simulink library "DblSlaveLib"  (R2020b)
settings: Solver=VariableStepAuto  StartTime=0.0  StopTime=10.0  RelTol=1e-3
libraries: simulink x7, InterpolationLib x4, $bdroot x3, Ramp_Library_R2017b x1
Description:
  | VLS Standard Library
  | Version: 1.0.0
settings Model: Creator=mchawa  LastModifiedBy=ahashem
settings DataIOCC: ReturnWorkspaceOutputs=off
settings DebuggingCC: ArithmeticOperatorsInVariantConditions=warning
settings SFSimCC: SimUseLocalCustomCode=off  CustomCodeUndefinedFunction=UseInterfaceOnly
settings RTWCC: RTWUseLocalCustomCode=off

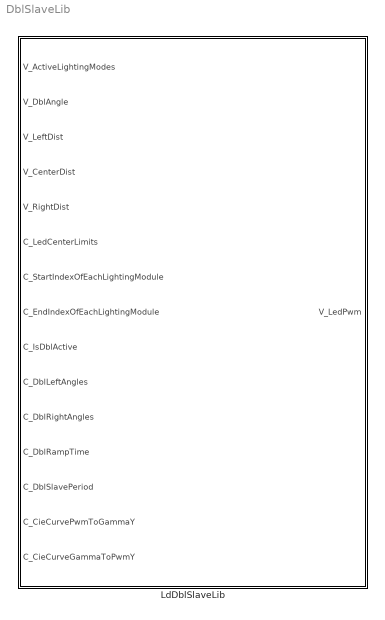
== system DblSlaveLib ==
  LdDblSlaveLib : Subsystem

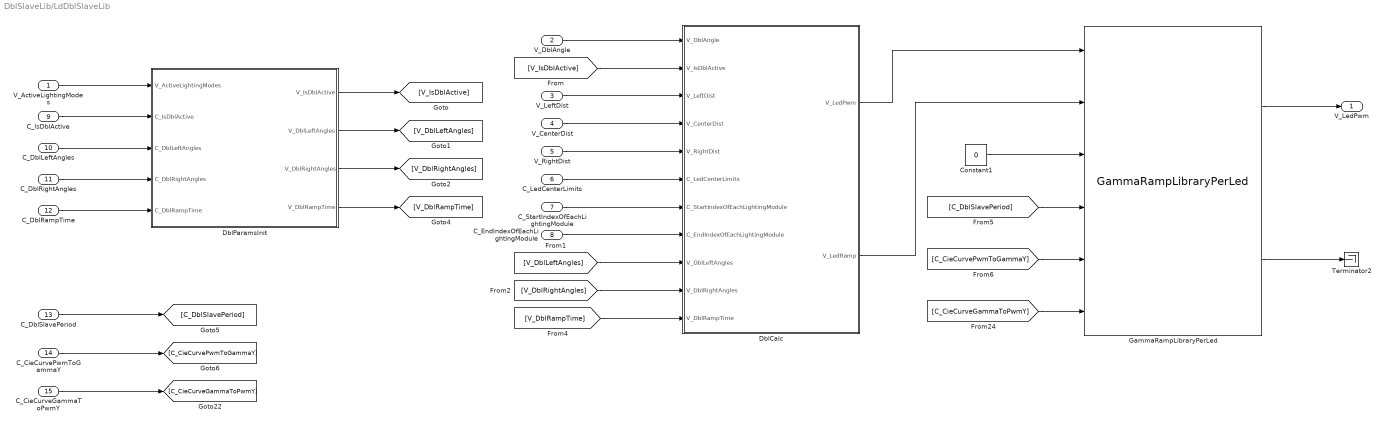
== system DblSlaveLib/LdDblSlaveLib ==
  V_ActiveLightingModes : Inport
  V_DblAngle : Inport  Port=2
  V_LeftDist : Inport  Port=3
  V_CenterDist : Inport  Port=4
  V_RightDist : Inport  Port=5
  C_LedCenterLimits : Inport  Port=6
  C_StartIndexOfEachLightingModule : Inport  Port=7
  C_EndIndexOfEachLightingModule : Inport  Port=8
  C_IsDblActive : Inport  Port=9
  C_DblLeftAngles : Inport  Port=10
  C_DblRightAngles : Inport  Port=11
  C_DblRampTime : Inport  Port=12
  C_DblSlavePeriod : Inport  Port=13
  C_CieCurvePwmToGammaY : Inport  Port=14
  C_CieCurveGammaToPwmY : Inport  Port=15
  Constant1 : Constant  Value=0  OutDataTypeStr=uint8
  DblCalc : Subsystem  TreatAsAtomicUnit=on
  DblParamsInit : Subsystem  TreatAsAtomicUnit=on
  GammaRampLibraryPerLed : Ramp_Library_R2017b/GammaRampLibraryPerLed  Description=|  SystemSampleTime=-1  VariantActivationTime=update diagram  Latency=0  AutoFrameSizeCalculation=off
      | This library performs ramp function taking CIE curves which are evenly distributed.
      | It performs the ramp linearly on the Gamma Curve.
  Terminator2 : Terminator
  V_LedPwm : Outport  VectorParamsAs1DForOutWhenUnconnected=off
  wires:
  C_EndIndexOfEachLightingModule/1 -> DblCalc/8(C_EndIndexOfEachLightingModule)
  DblParamsInit/1(V_IsDblActive) -> [V_IsDblActive]
  DblParamsInit/2(V_DblLeftAngles) -> [V_DblLeftAngles]
  [V_DblLeftAngles] -> DblCalc/9(V_DblLeftAngles)
  [V_DblRightAngles] -> DblCalc/10(V_DblRightAngles)
  C_LedCenterLimits/1 -> DblCalc/6(C_LedCenterLimits)
  DblParamsInit/3(V_DblRightAngles) -> [V_DblRightAngles]
  V_DblAngle/1 -> DblCalc/1(V_DblAngle)
  [V_IsDblActive] -> DblCalc/2(V_IsDblActive)
  C_StartIndexOfEachLightingModule/1 -> DblCalc/7(C_StartIndexOfEachLightingModule)
  GammaRampLibraryPerLed/1 -> V_LedPwm/1
  V_ActiveLightingModes/1 -> DblParamsInit/1(V_ActiveLightingModes)
  V_LeftDist/1 -> DblCalc/3(V_LeftDist)
  V_RightDist/1 -> DblCalc/5(V_RightDist)
  C_IsDblActive/1 -> DblParamsInit/2(C_IsDblActive)
  C_DblRampTime/1 -> DblParamsInit/5(C_DblRampTime)
  DblParamsInit/4(V_DblRampTime) -> [V_DblRampTime]
  C_DblLeftAngles/1 -> DblParamsInit/3(C_DblLeftAngles)
  V_CenterDist/1 -> DblCalc/4(V_CenterDist)
  C_DblRightAngles/1 -> DblParamsInit/4(C_DblRightAngles)
  DblCalc/1(V_LedPwm) -> GammaRampLibraryPerLed/1
  Constant1/1 -> GammaRampLibraryPerLed/3
  GammaRampLibraryPerLed/2 -> Terminator2/1
  C_CieCurveGammaToPwmY/1 -> [C_CieCurveGammaToPwmY]
  C_CieCurvePwmToGammaY/1 -> [C_CieCurvePwmToGammaY]
  C_DblSlavePeriod/1 -> [C_DblSlavePeriod]
  [C_CieCurveGammaToPwmY] -> GammaRampLibraryPerLed/6
  [C_CieCurvePwmToGammaY] -> GammaRampLibraryPerLed/5
  [C_DblSlavePeriod] -> GammaRampLibraryPerLed/4
  [V_DblRampTime] -> DblCalc/11(V_DblRampTime)
  DblCalc/2(V_LedRamp) -> GammaRampLibraryPerLed/2

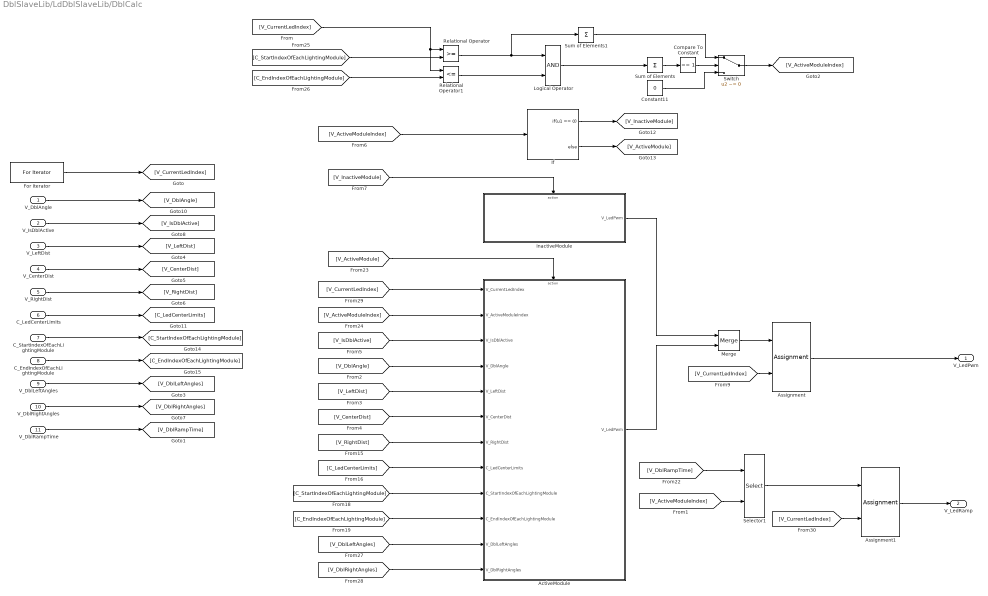
== system DblSlaveLib/LdDblSlaveLib/DblCalc ==
  V_DblAngle : Inport
  V_IsDblActive : Inport  Port=2
  V_LeftDist : Inport  Port=3
  V_CenterDist : Inport  Port=4
  V_RightDist : Inport  Port=5
  C_LedCenterLimits : Inport  Port=6
  C_StartIndexOfEachLightingModule : Inport  Port=7
  C_EndIndexOfEachLightingModule : Inport  Port=8
  V_DblLeftAngles : Inport  Port=9
  V_DblRightAngles : Inport  Port=10
  V_DblRampTime : Inport  Port=11
  ActiveModule : Subsystem  TreatAsAtomicUnit=on
  Assignment : Assignment  IndexMode=Zero-based  OutputInitialize=Specify size for each dimension in table  DiagnosticForDimensions=Error  IndexOptions=Index vector (port)  Indices=1  OutputSizes=C_NumOfLightingLeds
  Assignment1 : Assignment  IndexMode=Zero-based  OutputInitialize=Specify size for each dimension in table  DiagnosticForDimensions=Error  IndexOptions=Index vector (port)  Indices=1  OutputSizes=C_NumOfLightingLeds
  Compare To Constant : simulink/Logic and Bit Operations/Compare To Constant  relop===  const=1  OutDataTypeStr=boolean
  Constant11 : Constant  Value=0  OutDataTypeStr=Inherit: Inherit via back propagation
  For Iterator : ForIterator  IterationLimit=C_NumOfLightingLeds  IndexMode=Zero-based
  If : If  IfExpression=u1 == 0
  InactiveModule : Subsystem  TreatAsAtomicUnit=on
  Logical Operator : Logic  AllPortsSameDT=off  OutDataTypeStr=boolean
  Merge : Merge
  Relational Operator : RelationalOperator  OutDataTypeStr=boolean  RndMeth=Simplest
  Relational Operator1 : RelationalOperator  Operator=<=  OutDataTypeStr=boolean  RndMeth=Simplest
  Selector1 : Selector  IndexOptions=Index vector (port)  Indices=[1 3]  OutputSizes=1
  Sum of Elements : Sum  Inputs=+
  Sum of Elements1 : Sum  Inputs=+
  Switch : Switch  Criteria=u2 ~= 0
  V_LedPwm : Outport  VectorParamsAs1DForOutWhenUnconnected=off
  V_LedRamp : Outport  Port=2  VectorParamsAs1DForOutWhenUnconnected=off
  wires:
  For Iterator/1 -> [V_CurrentLedIndex]
  [V_CurrentLedIndex] -> Relational Operator/1, Relational Operator1/1
  V_LeftDist/1 -> [V_LeftDist]
  V_CenterDist/1 -> [V_CenterDist]
  V_RightDist/1 -> [V_RightDist]
  V_DblAngle/1 -> [V_DblAngle]
  Assignment/1 -> V_LedPwm/1
  [V_CurrentLedIndex] -> Assignment/2
  Relational Operator/1 -> Sum of Elements1/1, Logical Operator/1
  Logical Operator/1 -> Sum of Elements/1
  Relational Operator1/1 -> Logical Operator/2
  Sum of Elements/1 -> Compare To Constant/1
  Switch/1 -> [V_ActiveModuleIndex]
  Constant11/1 -> Switch/3
  Sum of Elements1/1 -> Switch/1
  Compare To Constant/1 -> Switch/2
  C_LedCenterLimits/1 -> [C_LedCenterLimits]
  [V_ActiveModuleIndex] -> If/1
  If/1 -> [V_InactiveModule]
  If/2 -> [V_ActiveModule]
  [V_InactiveModule] -> InactiveModule/Action
  [V_ActiveModule] -> ActiveModule/Action
  [V_ActiveModuleIndex] -> ActiveModule/2(V_ActiveModuleIndex)
  C_StartIndexOfEachLightingModule/1 -> [C_StartIndexOfEachLightingModule]
  C_EndIndexOfEachLightingModule/1 -> [C_EndIndexOfEachLightingModule]
  [C_StartIndexOfEachLightingModule] -> Relational Operator/2
  [C_EndIndexOfEachLightingModule] -> Relational Operator1/2
  ActiveModule/1(V_LedPwm) -> Merge/2
  InactiveModule/1(V_LedPwm) -> Merge/1
  Merge/1 -> Assignment/1
  V_DblLeftAngles/1 -> [V_DblLeftAngles]
  V_DblRightAngles/1 -> [V_DblRightAngles]
  [V_DblAngle] -> ActiveModule/4(V_DblAngle)
  [V_LeftDist] -> ActiveModule/5(V_LeftDist)
  [V_CenterDist] -> ActiveModule/6(V_CenterDist)
  [V_RightDist] -> ActiveModule/7(V_RightDist)
  [C_LedCenterLimits] -> ActiveModule/8(C_LedCenterLimits)
  [C_StartIndexOfEachLightingModule] -> ActiveModule/9(C_StartIndexOfEachLightingModule)
  [C_EndIndexOfEachLightingModule] -> ActiveModule/10(C_EndIndexOfEachLightingModule)
  [V_DblLeftAngles] -> ActiveModule/11(V_DblLeftAngles)
  [V_DblRightAngles] -> ActiveModule/12(V_DblRightAngles)
  [V_CurrentLedIndex] -> ActiveModule/1(V_CurrentLedIndex)
  V_IsDblActive/1 -> [V_IsDblActive]
  [V_IsDblActive] -> ActiveModule/3(V_IsDblActive)
  V_DblRampTime/1 -> [V_DblRampTime]
  Selector1/1 -> Assignment1/1
  [V_CurrentLedIndex] -> Assignment1/2
  Assignment1/1 -> V_LedRamp/1
  [V_DblRampTime] -> Selector1/1
  [V_ActiveModuleIndex] -> Selector1/2

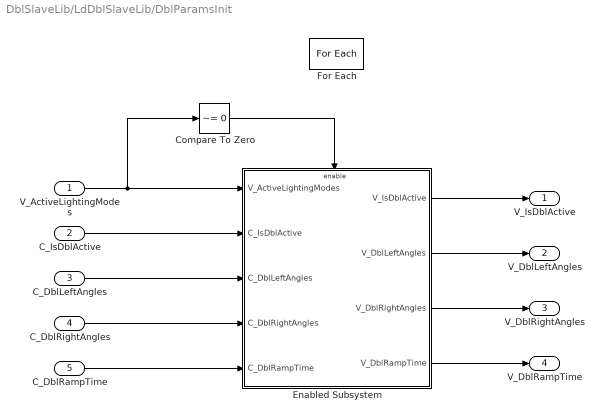
== system DblSlaveLib/LdDblSlaveLib/DblParamsInit ==
  V_ActiveLightingModes : Inport  Partition=on  PartitionDimension=1  PartitionWidth=1  PartitionOffset=0
  C_IsDblActive : Inport  Port=2  Partition=on  PartitionDimension=1  PartitionWidth=1  PartitionOffset=0
  C_DblLeftAngles : Inport  Port=3  Partition=on  PartitionDimension=1  PartitionWidth=1  PartitionOffset=0
  C_DblRightAngles : Inport  Port=4  Partition=on  PartitionDimension=1  PartitionWidth=1  PartitionOffset=0
  C_DblRampTime : Inport  Port=5  Partition=on  PartitionDimension=1  PartitionWidth=1  PartitionOffset=0
  Compare To Zero : simulink/Logic and Bit Operations/Compare To Zero  relop=~=  OutDataTypeStr=boolean
  Enabled Subsystem : Subsystem  TreatAsAtomicUnit=on
  For Each : ForEach  DisableCoverage=on
  V_IsDblActive : Outport  ConcatenationDimension=1  VectorParamsAs1DForOutWhenUnconnected=off
  V_DblLeftAngles : Outport  Port=2  ConcatenationDimension=1  VectorParamsAs1DForOutWhenUnconnected=off
  V_DblRightAngles : Outport  Port=3  ConcatenationDimension=1  VectorParamsAs1DForOutWhenUnconnected=off
  V_DblRampTime : Outport  Port=4  ConcatenationDimension=1  VectorParamsAs1DForOutWhenUnconnected=off
  wires:
  Compare To Zero/1 -> Enabled Subsystem/Enable
  V_ActiveLightingModes/1 -> Compare To Zero/1, Enabled Subsystem/1(V_ActiveLightingModes)
  C_IsDblActive/1 -> Enabled Subsystem/2(C_IsDblActive)
  Enabled Subsystem/1(V_IsDblActive) -> V_IsDblActive/1
  C_DblLeftAngles/1 -> Enabled Subsystem/3(C_DblLeftAngles)
  C_DblRightAngles/1 -> Enabled Subsystem/4(C_DblRightAngles)
  Enabled Subsystem/3(V_DblRightAngles) -> V_DblRightAngles/1
  Enabled Subsystem/2(V_DblLeftAngles) -> V_DblLeftAngles/1
  C_DblRampTime/1 -> Enabled Subsystem/5(C_DblRampTime)
  Enabled Subsystem/4(V_DblRampTime) -> V_DblRampTime/1

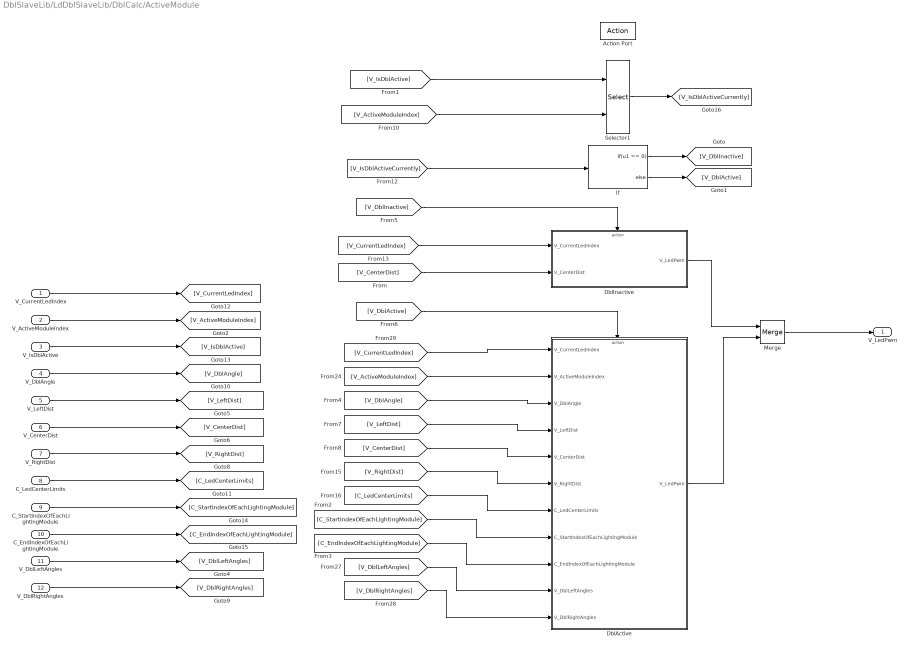
== system DblSlaveLib/LdDblSlaveLib/DblCalc/ActiveModule ==
  V_CurrentLedIndex : Inport
  V_ActiveModuleIndex : Inport  Port=2
  V_IsDblActive : Inport  Port=3
  V_DblAngle : Inport  Port=4
  V_LeftDist : Inport  Port=5
  V_CenterDist : Inport  Port=6
  V_RightDist : Inport  Port=7
  C_LedCenterLimits : Inport  Port=8
  C_StartIndexOfEachLightingModule : Inport  Port=9
  C_EndIndexOfEachLightingModule : Inport  Port=10
  V_DblLeftAngles : Inport  Port=11
  V_DblRightAngles : Inport  Port=12
  Action Port : ActionPort
  DblActive : Subsystem  TreatAsAtomicUnit=on
  DblInactive : Subsystem  TreatAsAtomicUnit=on
  If : If  IfExpression=u1 == 0
  Merge : Merge
  Selector1 : Selector  IndexOptions=Index vector (port)  Indices=[1 3]  OutputSizes=1
  V_LedPwm : Outport  VectorParamsAs1DForOutWhenUnconnected=off
  wires:
  [V_IsDblActiveCurrently] -> If/1
  If/1 -> [V_DblInactive]
  If/2 -> [V_DblActive]
  [V_DblInactive] -> DblInactive/Action
  [V_DblActive] -> DblActive/Action
  DblActive/1(V_LedPwm) -> Merge/2
  DblInactive/1(V_LedPwm) -> Merge/1
  Merge/1 -> V_LedPwm/1
  V_ActiveModuleIndex/1 -> [V_ActiveModuleIndex]
  V_DblAngle/1 -> [V_DblAngle]
  V_LeftDist/1 -> [V_LeftDist]
  V_CenterDist/1 -> [V_CenterDist]
  V_RightDist/1 -> [V_RightDist]
  C_LedCenterLimits/1 -> [C_LedCenterLimits]
  C_StartIndexOfEachLightingModule/1 -> [C_StartIndexOfEachLightingModule]
  C_EndIndexOfEachLightingModule/1 -> [C_EndIndexOfEachLightingModule]
  V_DblLeftAngles/1 -> [V_DblLeftAngles]
  V_DblRightAngles/1 -> [V_DblRightAngles]
  V_CurrentLedIndex/1 -> [V_CurrentLedIndex]
  [V_CurrentLedIndex] -> DblActive/1(V_CurrentLedIndex)
  [V_ActiveModuleIndex] -> DblActive/2(V_ActiveModuleIndex)
  [V_DblAngle] -> DblActive/3(V_DblAngle)
  [V_LeftDist] -> DblActive/4(V_LeftDist)
  [V_CenterDist] -> DblActive/5(V_CenterDist)
  [V_RightDist] -> DblActive/6(V_RightDist)
  [C_LedCenterLimits] -> DblActive/7(C_LedCenterLimits)
  [C_StartIndexOfEachLightingModule] -> DblActive/8(C_StartIndexOfEachLightingModule)
  [C_EndIndexOfEachLightingModule] -> DblActive/9(C_EndIndexOfEachLightingModule)
  [V_DblLeftAngles] -> DblActive/10(V_DblLeftAngles)
  [V_DblRightAngles] -> DblActive/11(V_DblRightAngles)
  V_IsDblActive/1 -> [V_IsDblActive]
  [V_IsDblActive] -> Selector1/1
  [V_ActiveModuleIndex] -> Selector1/2
  Selector1/1 -> [V_IsDblActiveCurrently]
  [V_CenterDist] -> DblInactive/2(V_CenterDist)
  [V_CurrentLedIndex] -> DblInactive/1(V_CurrentLedIndex)

== system DblSlaveLib/LdDblSlaveLib/DblCalc/InactiveModule ==
  Action Port : ActionPort
  Constant : Constant  Value=0  OutDataTypeStr=Inherit: Inherit via back propagation
  V_LedPwm : Outport  VectorParamsAs1DForOutWhenUnconnected=off
  wires:
  Constant/1 -> V_LedPwm/1

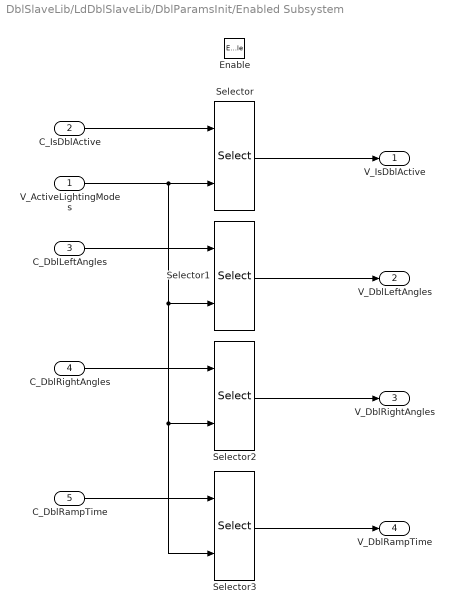
== system DblSlaveLib/LdDblSlaveLib/DblParamsInit/Enabled Subsystem ==
  V_ActiveLightingModes : Inport
  C_IsDblActive : Inport  Port=2
  C_DblLeftAngles : Inport  Port=3
  C_DblRightAngles : Inport  Port=4
  C_DblRampTime : Inport  Port=5
  Enable : EnablePort
  Selector{,1..3} (4 alike) : Selector  IndexOptions=Index vector (port)  Indices=[1 3]  OutputSizes=1
  V_IsDblActive : Outport  VectorParamsAs1DForOutWhenUnconnected=off
  V_DblLeftAngles : Outport  Port=2  VectorParamsAs1DForOutWhenUnconnected=off
  V_DblRightAngles : Outport  Port=3  VectorParamsAs1DForOutWhenUnconnected=off
  V_DblRampTime : Outport  Port=4  VectorParamsAs1DForOutWhenUnconnected=off
  wires:
  Selector/1 -> V_IsDblActive/1
  C_IsDblActive/1 -> Selector/1
  V_ActiveLightingModes/1 -> Selector3/2, Selector2/2, Selector1/2, Selector/2
  C_DblLeftAngles/1 -> Selector1/1
  C_DblRightAngles/1 -> Selector2/1
  Selector1/1 -> V_DblLeftAngles/1
  Selector2/1 -> V_DblRightAngles/1
  C_DblRampTime/1 -> Selector3/1
  Selector3/1 -> V_DblRampTime/1

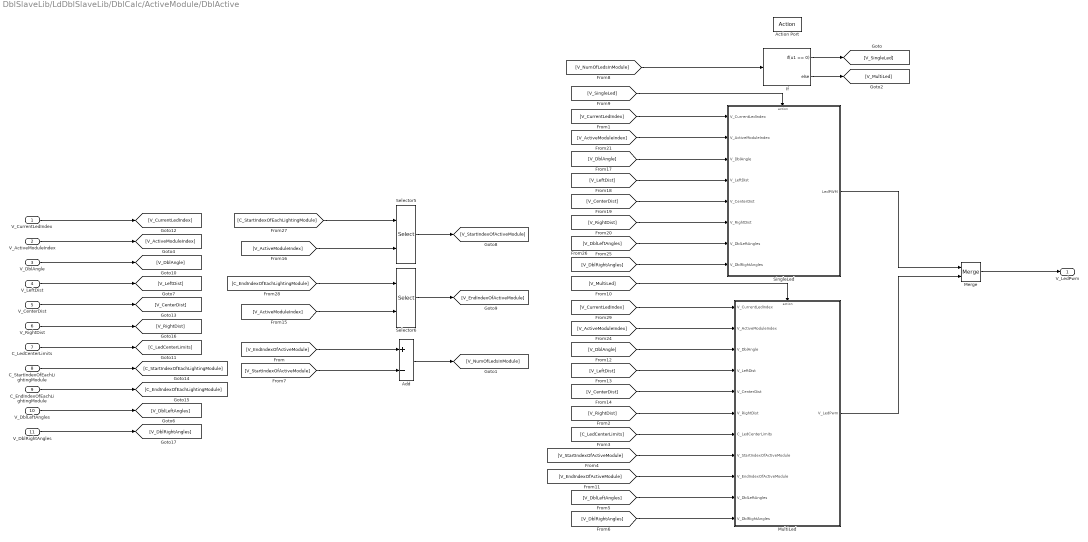
== system DblSlaveLib/LdDblSlaveLib/DblCalc/ActiveModule/DblActive ==
  V_CurrentLedIndex : Inport
  V_ActiveModuleIndex : Inport  Port=2
  V_DblAngle : Inport  Port=3
  V_LeftDist : Inport  Port=4
  V_CenterDist : Inport  Port=5
  V_RightDist : Inport  Port=6
  C_LedCenterLimits : Inport  Port=7
  C_StartIndexOfEachLightingModule : Inport  Port=8
  C_EndIndexOfEachLightingModule : Inport  Port=9
  V_DblLeftAngles : Inport  Port=10
  V_DblRightAngles : Inport  Port=11
  Action Port : ActionPort
  Add : Sum  Inputs=+-
  If : If  IfExpression=u1 == 0
  Merge : Merge
  MultiLed : Subsystem  TreatAsAtomicUnit=on
  Selector5 : Selector  IndexOptions=Index vector (port)  Indices=[1 3]  OutputSizes=1
  Selector6 : Selector  IndexOptions=Index vector (port)  Indices=[1 3]  OutputSizes=1
  SingleLed : Subsystem  TreatAsAtomicUnit=on
  V_LedPwm : Outport  VectorParamsAs1DForOutWhenUnconnected=off
  wires:
  [V_ActiveModuleIndex] -> Selector5/2
  [C_EndIndexOfEachLightingModule] -> Selector6/1
  [V_ActiveModuleIndex] -> Selector6/2
  Selector6/1 -> [V_EndIndexOfActiveModule]
  [C_StartIndexOfEachLightingModule] -> Selector5/1
  Selector5/1 -> [V_StartIndexOfActiveModule]
  [V_EndIndexOfActiveModule] -> Add/1
  [V_StartIndexOfActiveModule] -> Add/2
  Add/1 -> [V_NumOfLedsInModule]
  [V_NumOfLedsInModule] -> If/1
  If/1 -> [V_SingleLed]
  If/2 -> [V_MultiLed]
  [V_SingleLed] -> SingleLed/Action
  [V_MultiLed] -> MultiLed/Action
  MultiLed/1(V_LedPwm) -> Merge/2
  Merge/1 -> V_LedPwm/1
  V_CurrentLedIndex/1 -> [V_CurrentLedIndex]
  V_ActiveModuleIndex/1 -> [V_ActiveModuleIndex]
  V_DblAngle/1 -> [V_DblAngle]
  V_LeftDist/1 -> [V_LeftDist]
  V_CenterDist/1 -> [V_CenterDist]
  V_RightDist/1 -> [V_RightDist]
  C_LedCenterLimits/1 -> [C_LedCenterLimits]
  C_StartIndexOfEachLightingModule/1 -> [C_StartIndexOfEachLightingModule]
  C_EndIndexOfEachLightingModule/1 -> [C_EndIndexOfEachLightingModule]
  V_DblLeftAngles/1 -> [V_DblLeftAngles]
  V_DblRightAngles/1 -> [V_DblRightAngles]
  [V_CurrentLedIndex] -> MultiLed/1(V_CurrentLedIndex)
  [V_ActiveModuleIndex] -> MultiLed/2(V_ActiveModuleIndex)
  [V_LeftDist] -> MultiLed/4(V_LeftDist)
  [V_CenterDist] -> MultiLed/5(V_CenterDist)
  [V_RightDist] -> MultiLed/6(V_RightDist)
  [C_LedCenterLimits] -> MultiLed/7(C_LedCenterLimits)
  [V_StartIndexOfActiveModule] -> MultiLed/8(V_StartIndexOfActiveModule)
  [V_EndIndexOfActiveModule] -> MultiLed/9(V_EndIndexOfActiveModule)
  [V_DblLeftAngles] -> MultiLed/10(V_DblLeftAngles)
  [V_DblRightAngles] -> MultiLed/11(V_DblRightAngles)
  [V_DblAngle] -> MultiLed/3(V_DblAngle)
  [V_DblRightAngles] -> SingleLed/8(V_DblRightAngles)
  [V_LeftDist] -> SingleLed/4(V_LeftDist)
  [V_DblAngle] -> SingleLed/3(V_DblAngle)
  [V_DblLeftAngles] -> SingleLed/7(V_DblLeftAngles)
  [V_ActiveModuleIndex] -> SingleLed/2(V_ActiveModuleIndex)
  [V_RightDist] -> SingleLed/6(V_RightDist)
  [V_CenterDist] -> SingleLed/5(V_CenterDist)
  SingleLed/1(LedPWM) -> Merge/1
  [V_CurrentLedIndex] -> SingleLed/1(V_CurrentLedIndex)

== system DblSlaveLib/LdDblSlaveLib/DblCalc/ActiveModule/DblInactive ==
  V_CurrentLedIndex : Inport
  V_CenterDist : Inport  Port=2
  Action Port : ActionPort
  Selector : Selector  IndexMode=Zero-based  IndexOptions=Index vector (port)  Indices=[1 3]  OutputSizes=1
  V_LedPwm : Outport  VectorParamsAs1DForOutWhenUnconnected=off
  wires:
  V_CenterDist/1 -> Selector/1
  V_CurrentLedIndex/1 -> Selector/2
  Selector/1 -> V_LedPwm/1

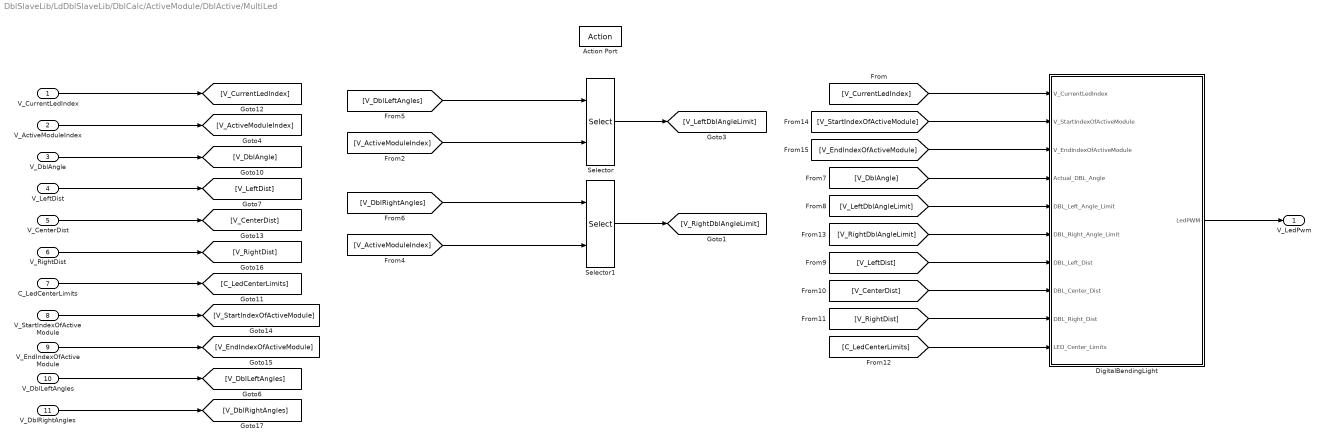
== system DblSlaveLib/LdDblSlaveLib/DblCalc/ActiveModule/DblActive/MultiLed ==
  V_CurrentLedIndex : Inport
  V_ActiveModuleIndex : Inport  Port=2
  V_DblAngle : Inport  Port=3
  V_LeftDist : Inport  Port=4
  V_CenterDist : Inport  Port=5
  V_RightDist : Inport  Port=6
  C_LedCenterLimits : Inport  Port=7
  V_StartIndexOfActiveModule : Inport  Port=8
  V_EndIndexOfActiveModule : Inport  Port=9
  V_DblLeftAngles : Inport  Port=10
  V_DblRightAngles : Inport  Port=11
  Action Port : ActionPort
  DigitalBendingLight : Subsystem  Description=|  TreatAsAtomicUnit=on
      | This block performs DBL function assuming that the DBL Left/Center/Right Distribution are of the same size as LED_Center_Limits.
      | Left DBL_Angles must be always less than Right DBL_Angles.
  Selector : Selector  IndexOptions=Index vector (port)  Indices=[1 3]  OutputSizes=1
  Selector1 : Selector  IndexOptions=Index vector (port)  Indices=[1 3]  OutputSizes=1
  V_LedPwm : Outport  VectorParamsAs1DForOutWhenUnconnected=off
  wires:
  [V_ActiveModuleIndex] -> Selector1/2
  [V_DblRightAngles] -> Selector1/1
  [V_DblLeftAngles] -> Selector/1
  [V_ActiveModuleIndex] -> Selector/2
  DigitalBendingLight/1(LedPWM) -> V_LedPwm/1
  V_ActiveModuleIndex/1 -> [V_ActiveModuleIndex]
  V_DblAngle/1 -> [V_DblAngle]
  V_DblLeftAngles/1 -> [V_DblLeftAngles]
  V_RightDist/1 -> [V_RightDist]
  V_DblRightAngles/1 -> [V_DblRightAngles]
  V_EndIndexOfActiveModule/1 -> [V_EndIndexOfActiveModule]
  V_LeftDist/1 -> [V_LeftDist]
  V_StartIndexOfActiveModule/1 -> [V_StartIndexOfActiveModule]
  C_LedCenterLimits/1 -> [C_LedCenterLimits]
  V_CurrentLedIndex/1 -> [V_CurrentLedIndex]
  V_CenterDist/1 -> [V_CenterDist]
  [V_CurrentLedIndex] -> DigitalBendingLight/1(V_CurrentLedIndex)
  [V_DblAngle] -> DigitalBendingLight/4(Actual_DBL_Angle)
  [V_LeftDblAngleLimit] -> DigitalBendingLight/5(DBL_Left_Angle_Limit)
  [V_LeftDist] -> DigitalBendingLight/7(DBL_Left_Dist)
  [V_CenterDist] -> DigitalBendingLight/8(DBL_Center_Dist)
  [V_RightDist] -> DigitalBendingLight/9(DBL_Right_Dist)
  [C_LedCenterLimits] -> DigitalBendingLight/10(LED_Center_Limits)
  Selector/1 -> [V_LeftDblAngleLimit]
  Selector1/1 -> [V_RightDblAngleLimit]
  [V_RightDblAngleLimit] -> DigitalBendingLight/6(DBL_Right_Angle_Limit)
  [V_StartIndexOfActiveModule] -> DigitalBendingLight/2(V_StartIndexOfActiveModule)
  [V_EndIndexOfActiveModule] -> DigitalBendingLight/3(V_EndIndexOfActiveModule)

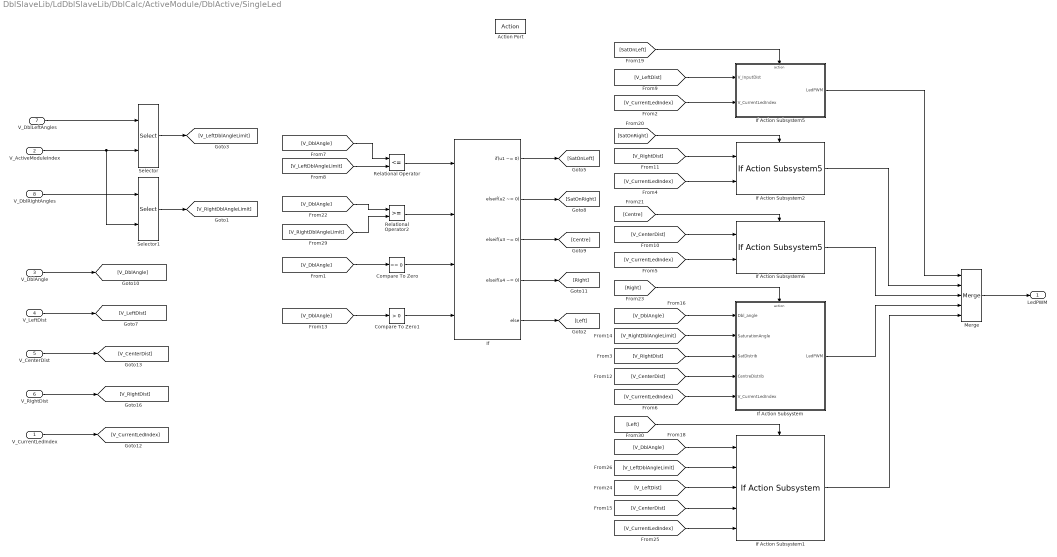
== system DblSlaveLib/LdDblSlaveLib/DblCalc/ActiveModule/DblActive/SingleLed ==
  V_CurrentLedIndex : Inport
  V_ActiveModuleIndex : Inport  Port=2
  V_DblAngle : Inport  Port=3
  V_LeftDist : Inport  Port=4
  V_CenterDist : Inport  Port=5
  V_RightDist : Inport  Port=6
  V_DblLeftAngles : Inport  Port=7
  V_DblRightAngles : Inport  Port=8
  Action Port : ActionPort
  Compare To Zero : simulink/Logic and Bit Operations/Compare To Zero  relop===  OutDataTypeStr=boolean
  Compare To Zero1 : simulink/Logic and Bit Operations/Compare To Zero  relop=>  OutDataTypeStr=boolean
  If : If  NumInputs=4  IfExpression=u1 ~= 0  ElseIfExpressions=u2 ~= 0, u3 ~= 0,u4 ~= 0
  If Action Subsystem : Subsystem  TreatAsAtomicUnit=on
  If Action Subsystem1 : $bdroot/LdDblSlaveLib/DblCalc/ActiveModule/DblActive/SingleLed/If Action Subsystem  SystemSampleTime=-1  VariantActivationTime=update diagram  Latency=0  AutoFrameSizeCalculation=off
  If Action Subsystem2 : $bdroot/LdDblSlaveLib/DblCalc/ActiveModule/DblActive/SingleLed/If Action Subsystem5  SystemSampleTime=-1  VariantActivationTime=update diagram  Latency=0  AutoFrameSizeCalculation=off
  If Action Subsystem5 : Subsystem  TreatAsAtomicUnit=on
  If Action Subsystem6 : $bdroot/LdDblSlaveLib/DblCalc/ActiveModule/DblActive/SingleLed/If Action Subsystem5  SystemSampleTime=-1  VariantActivationTime=update diagram  Latency=0  AutoFrameSizeCalculation=off
  Merge : Merge  Inputs=5  InitialOutput=0
  Relational Operator : RelationalOperator  Operator=<=  OutDataTypeStr=boolean  RndMeth=Simplest
  Relational Operator2 : RelationalOperator  OutDataTypeStr=boolean  RndMeth=Simplest
  Selector : Selector  IndexOptions=Index vector (port)  Indices=[1 3]  OutputSizes=1
  Selector1 : Selector  IndexOptions=Index vector (port)  Indices=[1 3]  OutputSizes=1
  LedPWM : Outport  VectorParamsAs1DForOutWhenUnconnected=off
  wires:
  V_DblRightAngles/1 -> Selector1/1
  V_DblLeftAngles/1 -> Selector/1
  Selector1/1 -> [V_RightDblAngleLimit]
  Selector/1 -> [V_LeftDblAngleLimit]
  V_ActiveModuleIndex/1 -> Selector/2, Selector1/2
  V_DblAngle/1 -> [V_DblAngle]
  V_LeftDist/1 -> [V_LeftDist]
  V_RightDist/1 -> [V_RightDist]
  V_CenterDist/1 -> [V_CenterDist]
  Relational Operator2/1 -> If/2
  Compare To Zero/1 -> If/3
  If/3 -> [Centre]
  [SatOnLeft] -> If Action Subsystem5/Action
  [V_CenterDist] -> If Action Subsystem6/1
  [Centre] -> If Action Subsystem6/Action
  Merge/1 -> LedPWM/1
  If/2 -> [SatOnRight]
  If/1 -> [SatOnLeft]
  Relational Operator/1 -> If/1
  [V_DblAngle] -> Compare To Zero/1
  [Right] -> If Action Subsystem/Action
  [V_DblAngle] -> Relational Operator2/1
  If/5 -> [Left]
  [V_RightDblAngleLimit] -> Relational Operator2/2
  [V_LeftDblAngleLimit] -> Relational Operator/2
  [V_DblAngle] -> Relational Operator/1
  Compare To Zero1/1 -> If/4
  [V_DblAngle] -> Compare To Zero1/1
  If/4 -> [Right]
  [Left] -> If Action Subsystem1/Action
  [V_RightDist] -> If Action Subsystem/3(SatDistrib)
  [V_CenterDist] -> If Action Subsystem/4(CentreDistrib)
  [V_RightDblAngleLimit] -> If Action Subsystem/2(SaturationAngle)
  [SatOnRight] -> If Action Subsystem2/Action
  [V_RightDist] -> If Action Subsystem2/1
  [V_DblAngle] -> If Action Subsystem/1(Dbl_angle)
  [V_DblAngle] -> If Action Subsystem1/1
  [V_LeftDblAngleLimit] -> If Action Subsystem1/2
  [V_CenterDist] -> If Action Subsystem1/4
  [V_LeftDist] -> If Action Subsystem1/3
  If Action Subsystem5/1(LedPWM) -> Merge/1
  If Action Subsystem2/1 -> Merge/2
  If Action Subsystem6/1 -> Merge/3
  If Action Subsystem/1(LedPWM) -> Merge/4
  If Action Subsystem1/1 -> Merge/5
  [V_LeftDist] -> If Action Subsystem5/1(V_InputDist)
  [V_CurrentLedIndex] -> If Action Subsystem5/2(V_CurrentLedIndex)
  V_CurrentLedIndex/1 -> [V_CurrentLedIndex]
  [V_CurrentLedIndex] -> If Action Subsystem2/2
  [V_CurrentLedIndex] -> If Action Subsystem6/2
  [V_CurrentLedIndex] -> If Action Subsystem/5(V_CurrentLedIndex)
  [V_CurrentLedIndex] -> If Action Subsystem1/5

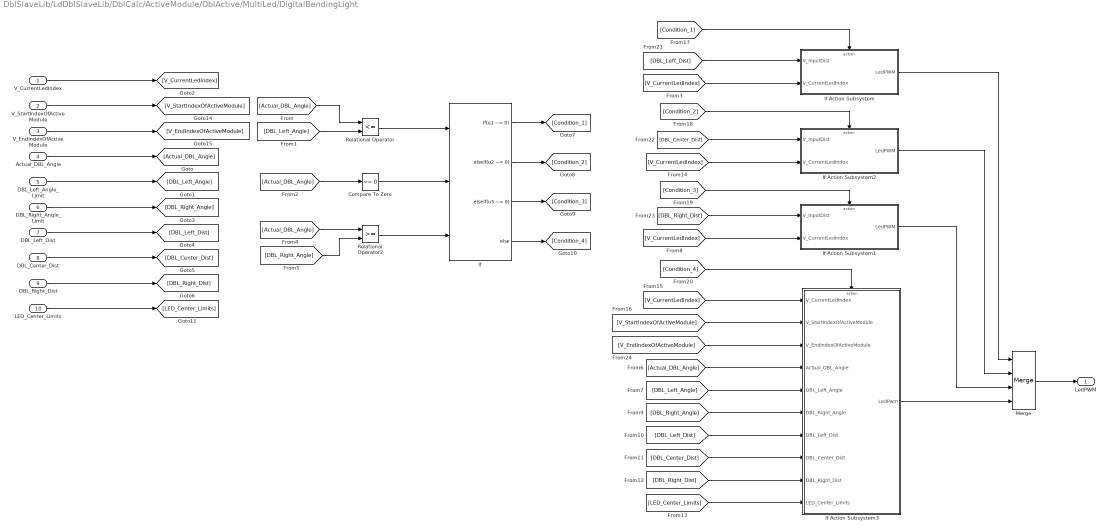
== system DblSlaveLib/LdDblSlaveLib/DblCalc/ActiveModule/DblActive/MultiLed/DigitalBendingLight ==
  V_CurrentLedIndex : Inport
  V_StartIndexOfActiveModule : Inport  Port=2
  V_EndIndexOfActiveModule : Inport  Port=3
  Actual_DBL_Angle : Inport  Port=4
  DBL_Left_Angle_Limit : Inport  Port=5
  DBL_Right_Angle_Limit : Inport  Port=6
  DBL_Left_Dist : Inport  Port=7
  DBL_Center_Dist : Inport  Port=8
  DBL_Right_Dist : Inport  Port=9
  LED_Center_Limits : Inport  Port=10
  Compare To Zero : simulink/Logic and Bit Operations/Compare To Zero  relop===  OutDataTypeStr=boolean
  If : If  NumInputs=3  IfExpression=u1 ~= 0  ElseIfExpressions=u2 ~= 0, u3 ~= 0
  If Action Subsystem : Subsystem  TreatAsAtomicUnit=on
  If Action Subsystem1 : Subsystem  TreatAsAtomicUnit=on
  If Action Subsystem2 : Subsystem  TreatAsAtomicUnit=on
  If Action Subsystem3 : Subsystem  TreatAsAtomicUnit=on
  Merge : Merge  Inputs=4  InitialOutput=0
  Relational Operator : RelationalOperator  Operator=<=  OutDataTypeStr=boolean  RndMeth=Simplest
  Relational Operator2 : RelationalOperator  OutDataTypeStr=boolean  RndMeth=Simplest
  LedPWM : Outport  VectorParamsAs1DForOutWhenUnconnected=off
  wires:
  Actual_DBL_Angle/1 -> [Actual_DBL_Angle]
  DBL_Left_Angle_Limit/1 -> [DBL_Left_Angle]
  DBL_Right_Angle_Limit/1 -> [DBL_Right_Angle]
  [Actual_DBL_Angle] -> Relational Operator/1
  [DBL_Left_Angle] -> Relational Operator/2
  [DBL_Right_Angle] -> Relational Operator2/2
  [Actual_DBL_Angle] -> Relational Operator2/1
  DBL_Left_Dist/1 -> [DBL_Left_Dist]
  DBL_Center_Dist/1 -> [DBL_Center_Dist]
  DBL_Right_Dist/1 -> [DBL_Right_Dist]
  Relational Operator/1 -> If/1
  [Actual_DBL_Angle] -> Compare To Zero/1
  Relational Operator2/1 -> If/3
  If/1 -> [Condition_1]
  If/2 -> [Condition_2]
  If/3 -> [Condition_3]
  [Condition_1] -> If Action Subsystem/Action
  [Condition_4] -> If Action Subsystem3/Action
  [DBL_Left_Dist] -> If Action Subsystem/1(V_InputDist)
  If/4 -> [Condition_4]
  [Actual_DBL_Angle] -> If Action Subsystem3/4(Actual_DBL_Angle)
  [DBL_Left_Angle] -> If Action Subsystem3/5(DBL_Left_Angle)
  [DBL_Right_Angle] -> If Action Subsystem3/6(DBL_Right_Angle)
  [DBL_Left_Dist] -> If Action Subsystem3/7(DBL_Left_Dist)
  [DBL_Center_Dist] -> If Action Subsystem3/8(DBL_Center_Dist)
  If Action Subsystem1/1(LedPWM) -> Merge/3
  If Action Subsystem2/1(LedPWM) -> Merge/2
  If Action Subsystem/1(LedPWM) -> Merge/1
  Merge/1 -> LedPWM/1
  [DBL_Right_Dist] -> If Action Subsystem3/9(DBL_Right_Dist)
  LED_Center_Limits/1 -> [LED_Center_Limits]
  [LED_Center_Limits] -> If Action Subsystem3/10(LED_Center_Limits)
  Compare To Zero/1 -> If/2
  V_CurrentLedIndex/1 -> [V_CurrentLedIndex]
  [V_CurrentLedIndex] -> If Action Subsystem/2(V_CurrentLedIndex)
  [DBL_Right_Dist] -> If Action Subsystem1/1(V_InputDist)
  [V_CurrentLedIndex] -> If Action Subsystem1/2(V_CurrentLedIndex)
  [Condition_3] -> If Action Subsystem1/Action
  [DBL_Center_Dist] -> If Action Subsystem2/1(V_InputDist)
  [V_CurrentLedIndex] -> If Action Subsystem2/2(V_CurrentLedIndex)
  [Condition_2] -> If Action Subsystem2/Action
  [V_CurrentLedIndex] -> If Action Subsystem3/1(V_CurrentLedIndex)
  V_StartIndexOfActiveModule/1 -> [V_StartIndexOfActiveModule]
  V_EndIndexOfActiveModule/1 -> [V_EndIndexOfActiveModule]
  [V_StartIndexOfActiveModule] -> If Action Subsystem3/2(V_StartIndexOfActiveModule)
  [V_EndIndexOfActiveModule] -> If Action Subsystem3/3(V_EndIndexOfActiveModule)
  If Action Subsystem3/1(LedPwm) -> Merge/4

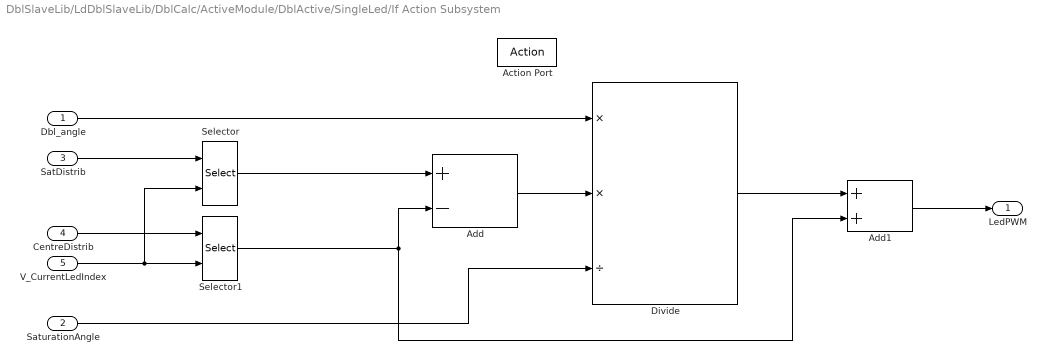
== system DblSlaveLib/LdDblSlaveLib/DblCalc/ActiveModule/DblActive/SingleLed/If Action Subsystem ==
  Dbl_angle : Inport
  SaturationAngle : Inport  Port=2
  SatDistrib : Inport  Port=3
  CentreDistrib : Inport  Port=4
  V_CurrentLedIndex : Inport  Port=5
  Action Port : ActionPort  ActionPortLabel=elseif(u4 ~= 0)
  Add : Sum  Inputs=+-  OutDataTypeStr=fixdt(1,16,0.1,0)
  Add1 : Sum  OutDataTypeStr=fixdt(0,16,0.01,0)
  Divide : Product  Inputs=**/  OutDataTypeStr=fixdt(1,16,0.1,0)
  Selector : Selector  IndexMode=Zero-based  IndexOptions=Index vector (port)  Indices=[1 3]  OutputSizes=1
  Selector1 : Selector  IndexMode=Zero-based  IndexOptions=Index vector (port)  Indices=[1 3]  OutputSizes=1
  LedPWM : Outport  VectorParamsAs1DForOutWhenUnconnected=off
  wires:
  Dbl_angle/1 -> Divide/1
  Selector1/1 -> Add/2, Add1/2
  Selector/1 -> Add/1
  SaturationAngle/1 -> Divide/3
  Add/1 -> Divide/2
  Divide/1 -> Add1/1
  V_CurrentLedIndex/1 -> Selector/2, Selector1/2
  Add1/1 -> LedPWM/1
  SatDistrib/1 -> Selector/1
  CentreDistrib/1 -> Selector1/1

== system DblSlaveLib/LdDblSlaveLib/DblCalc/ActiveModule/DblActive/SingleLed/If Action Subsystem5 ==
  V_InputDist : Inport
  V_CurrentLedIndex : Inport  Port=2
  Action Port : ActionPort  ActionPortLabel=if(u1 ~= 0)
  Selector : Selector  IndexMode=Zero-based  IndexOptions=Index vector (port)  Indices=[1 3]  OutputSizes=1
  LedPWM : Outport  VectorParamsAs1DForOutWhenUnconnected=off
  wires:
  V_CurrentLedIndex/1 -> Selector/2
  Selector/1 -> LedPWM/1
  V_InputDist/1 -> Selector/1

== system DblSlaveLib/LdDblSlaveLib/DblCalc/ActiveModule/DblActive/MultiLed/DigitalBendingLight/If Action Subsystem ==
  V_InputDist : Inport
  V_CurrentLedIndex : Inport  Port=2
  Action Port : ActionPort
  Selector : Selector  IndexMode=Zero-based  IndexOptions=Index vector (port)  Indices=[1 3]  OutputSizes=1
  LedPWM : Outport  VectorParamsAs1DForOutWhenUnconnected=off
  wires:
  V_InputDist/1 -> Selector/1
  V_CurrentLedIndex/1 -> Selector/2
  Selector/1 -> LedPWM/1

== system DblSlaveLib/LdDblSlaveLib/DblCalc/ActiveModule/DblActive/MultiLed/DigitalBendingLight/If Action Subsystem1 ==
  V_InputDist : Inport
  V_CurrentLedIndex : Inport  Port=2
  Action Port : ActionPort
  Selector : Selector  IndexMode=Zero-based  IndexOptions=Index vector (port)  Indices=[1 3]  OutputSizes=1
  LedPWM : Outport  VectorParamsAs1DForOutWhenUnconnected=off
  wires:
  Selector/1 -> LedPWM/1
  V_CurrentLedIndex/1 -> Selector/2
  V_InputDist/1 -> Selector/1

== system DblSlaveLib/LdDblSlaveLib/DblCalc/ActiveModule/DblActive/MultiLed/DigitalBendingLight/If Action Subsystem2 ==
  V_InputDist : Inport
  V_CurrentLedIndex : Inport  Port=2
  Action Port : ActionPort
  Selector : Selector  IndexMode=Zero-based  IndexOptions=Index vector (port)  Indices=[1 3]  OutputSizes=1
  LedPWM : Outport  VectorParamsAs1DForOutWhenUnconnected=off
  wires:
  V_InputDist/1 -> Selector/1
  V_CurrentLedIndex/1 -> Selector/2
  Selector/1 -> LedPWM/1

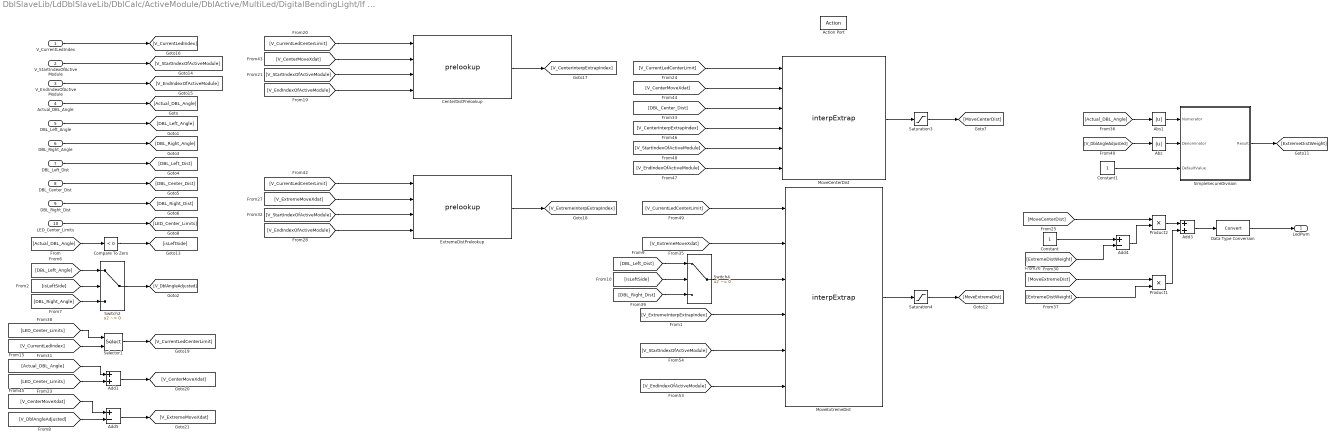
== system DblSlaveLib/LdDblSlaveLib/DblCalc/ActiveModule/DblActive/MultiLed/DigitalBendingLight/If Action Subsystem3 ==
  V_CurrentLedIndex : Inport
  V_StartIndexOfActiveModule : Inport  Port=2
  V_EndIndexOfActiveModule : Inport  Port=3
  Actual_DBL_Angle : Inport  Port=4
  DBL_Left_Angle : Inport  Port=5
  DBL_Right_Angle : Inport  Port=6
  DBL_Left_Dist : Inport  Port=7
  DBL_Center_Dist : Inport  Port=8
  DBL_Right_Dist : Inport  Port=9
  LED_Center_Limits : Inport  Port=10
  Action Port : ActionPort
  Abs : Abs
  Abs1 : Abs
  Add1 : Sum
  Add3 : Sum  OutDataTypeStr=Inherit: Inherit via back propagation
  Add4 : Sum  Inputs=+-  OutDataTypeStr=fixdt(1,16,0.001,0)  RndMeth=Nearest
  Add5 : Sum  Inputs=+-
  CenterDistPrelookup : InterpolationLib/prelookup  SystemSampleTime=-1  VariantActivationTime=update diagram  Latency=0  AutoFrameSizeCalculation=off
  Compare To Zero : simulink/Logic and Bit Operations/Compare To Zero  relop=<  OutDataTypeStr=boolean
  Constant : Constant  OutDataTypeStr=uint8
  Constant1 : Constant  OutDataTypeStr=fixdt(1,16,0.001,0)
  Data Type Conversion : DataTypeConversion
  ExtremeDistPrelookup : InterpolationLib/prelookup  SystemSampleTime=-1  VariantActivationTime=update diagram  Latency=0  AutoFrameSizeCalculation=off
  MoveCenterDist : InterpolationLib/interpExtrap  SystemSampleTime=-1  VariantActivationTime=update diagram  Latency=0  AutoFrameSizeCalculation=off
  MoveExtremeDist : InterpolationLib/interpExtrap  SystemSampleTime=-1  VariantActivationTime=update diagram  Latency=0  AutoFrameSizeCalculation=off
  Product1 : Product  OutDataTypeStr=Inherit: Same as first input
  Product2 : Product  OutDataTypeStr=Inherit: Same as first input
  Saturation3 : Saturate  UpperLimit=100  LowerLimit=0  OutDataTypeStr=Inherit: Inherit via back propagation
  Saturation4 : Saturate  UpperLimit=100  LowerLimit=0  OutDataTypeStr=Inherit: Inherit via back propagation
  Selector1 : Selector  IndexMode=Zero-based  IndexOptions=Index vector (port)  Indices=[1 3]  OutputSizes=1
  SimpleSecureDivision : Subsystem
  Switch2 : Switch  Criteria=u2 ~= 0
  Switch4 : Switch  Criteria=u2 ~= 0
  LedPwm : Outport  VectorParamsAs1DForOutWhenUnconnected=off
  wires:
  DBL_Left_Angle/1 -> [DBL_Left_Angle]
  DBL_Right_Angle/1 -> [DBL_Right_Angle]
  DBL_Left_Dist/1 -> [DBL_Left_Dist]
  DBL_Center_Dist/1 -> [DBL_Center_Dist]
  DBL_Right_Dist/1 -> [DBL_Right_Dist]
  LED_Center_Limits/1 -> [LED_Center_Limits]
  [MoveExtremeDist] -> Product1/1
  Product1/1 -> Add3/2
  Product2/1 -> Add3/1
  [MoveCenterDist] -> Product2/1
  [ExtremeDistWeight] -> Product1/2
  Actual_DBL_Angle/1 -> [Actual_DBL_Angle]
  [V_DblAngleAdjusted] -> Abs/1
  Abs/1 -> SimpleSecureDivision/2(Denominator)
  Abs1/1 -> SimpleSecureDivision/1(Numerator)
  [Actual_DBL_Angle] -> Abs1/1
  SimpleSecureDivision/1(Result) -> [ExtremeDistWeight]
  Add4/1 -> Product2/2
  [ExtremeDistWeight] -> Add4/2
  Constant/1 -> Add4/1
  Add3/1 -> Data Type Conversion/1
  Constant1/1 -> SimpleSecureDivision/3(DefaultValue)
  Data Type Conversion/1 -> LedPwm/1
  [Actual_DBL_Angle] -> Compare To Zero/1
  Compare To Zero/1 -> [isLeftSide]
  [DBL_Right_Angle] -> Switch2/3
  [DBL_Left_Angle] -> Switch2/1
  [isLeftSide] -> Switch2/2
  V_EndIndexOfActiveModule/1 -> [V_EndIndexOfActiveModule]
  V_StartIndexOfActiveModule/1 -> [V_StartIndexOfActiveModule]
  V_CurrentLedIndex/1 -> [V_CurrentLedIndex]
  [V_StartIndexOfActiveModule] -> CenterDistPrelookup/3
  [V_EndIndexOfActiveModule] -> CenterDistPrelookup/4
  CenterDistPrelookup/1 -> [V_CenterInterpExtrapIndex]
  ExtremeDistPrelookup/1 -> [V_ExtremeInterpExtrapIndex]
  Switch2/1 -> [V_DblAngleAdjusted]
  [V_StartIndexOfActiveModule] -> ExtremeDistPrelookup/3
  [V_EndIndexOfActiveModule] -> ExtremeDistPrelookup/4
  [LED_Center_Limits] -> Selector1/1
  [V_CurrentLedIndex] -> Selector1/2
  MoveCenterDist/1 -> Saturation3/1
  Selector1/1 -> [V_CurrentLedCenterLimit]
  [V_CurrentLedCenterLimit] -> ExtremeDistPrelookup/1
  [V_CurrentLedCenterLimit] -> CenterDistPrelookup/1
  [V_CurrentLedCenterLimit] -> MoveCenterDist/1
  [V_CenterMoveXdat] -> CenterDistPrelookup/2
  [V_CenterMoveXdat] -> MoveCenterDist/2
  [V_ExtremeMoveXdat] -> ExtremeDistPrelookup/2
  [DBL_Center_Dist] -> MoveCenterDist/3
  [V_CenterInterpExtrapIndex] -> MoveCenterDist/4
  [V_StartIndexOfActiveModule] -> MoveCenterDist/5
  [V_EndIndexOfActiveModule] -> MoveCenterDist/6
  Saturation3/1 -> [MoveCenterDist]
  [V_CurrentLedCenterLimit] -> MoveExtremeDist/1
  [V_ExtremeMoveXdat] -> MoveExtremeDist/2
  Switch4/1 -> MoveExtremeDist/3
  [V_ExtremeInterpExtrapIndex] -> MoveExtremeDist/4
  [V_StartIndexOfActiveModule] -> MoveExtremeDist/5
  [V_EndIndexOfActiveModule] -> MoveExtremeDist/6
  Saturation4/1 -> [MoveExtremeDist]
  MoveExtremeDist/1 -> Saturation4/1
  [DBL_Left_Dist] -> Switch4/1
  [isLeftSide] -> Switch4/2
  [DBL_Right_Dist] -> Switch4/3
  Add1/1 -> [V_CenterMoveXdat]
  [V_CenterMoveXdat] -> Add5/1
  Add5/1 -> [V_ExtremeMoveXdat]
  [LED_Center_Limits] -> Add1/2
  [V_DblAngleAdjusted] -> Add5/2
  [Actual_DBL_Angle] -> Add1/1

== system DblSlaveLib/LdDblSlaveLib/DblCalc/ActiveModule/DblActive/MultiLed/DigitalBendingLight/If Action Subsystem3/SimpleSecureDivision ==
  Numerator : Inport
  Denominator : Inport  Port=2
  DefaultValue : Inport  Port=3
  Compare To Zero : simulink/Logic and Bit Operations/Compare To Zero  relop=~=  OutDataTypeStr=boolean
  If : If  IfExpression=u1 ~= 0
  If Action Subsystem : Subsystem  TreatAsAtomicUnit=on
  If Action Subsystem1 : Subsystem  TreatAsAtomicUnit=on
  Merge : Merge  InitialOutput=1
  Result : Outport  VectorParamsAs1DForOutWhenUnconnected=off
  wires:
  Numerator/1 -> If Action Subsystem/1(Numerator)
  If/2 -> If Action Subsystem1/Action
  Denominator/1 -> If Action Subsystem/2(Denominator), Compare To Zero/1
  If Action Subsystem/1(Result) -> Merge/1
  If Action Subsystem1/1(Result) -> Merge/2
  Merge/1 -> Result/1
  DefaultValue/1 -> If Action Subsystem1/1(DefaultValue)
  If/1 -> If Action Subsystem/Action
  Compare To Zero/1 -> If/1

== system DblSlaveLib/LdDblSlaveLib/DblCalc/ActiveModule/DblActive/MultiLed/DigitalBendingLight/If Action Subsystem3/SimpleSecureDivision/If Action Subsystem ==
  Numerator : Inport
  Denominator : Inport  Port=2
  Action Port : ActionPort
  Divide : Product  Inputs=*/  OutDataTypeStr=Inherit: Inherit via back propagation
  Result : Outport  VectorParamsAs1DForOutWhenUnconnected=off
  wires:
  Divide/1 -> Result/1
  Numerator/1 -> Divide/1
  Denominator/1 -> Divide/2

== system DblSlaveLib/LdDblSlaveLib/DblCalc/ActiveModule/DblActive/MultiLed/DigitalBendingLight/If Action Subsystem3/SimpleSecureDivision/If Action Subsystem1 ==
  DefaultValue : Inport
  Action Port : ActionPort
  Result : Outport  VectorParamsAs1DForOutWhenUnconnected=off
  wires:
  DefaultValue/1 -> Result/1
